simulink model "single_phase_converter_i_pr_closeloop"  (R2022b)
settings: Solver=VariableStepAuto  StartTime=0.0  StopTime=0.1  FixedStep=1e-6  MaxStep=1e-8  RelTol=1e-7
model workspace (MAT data in the model file):
  Kp = 0.2
  Kr = 10
  Ts = 2.5e-05
  wc = 6.28318530718
  wr = 314.159265359
libraries: spsMosfetLib x4, spsSeriesRLCBranchLib x4, spsCurrentMeasurementLib x1, spsDCVoltageSourceLib x1, spsIdealSwitchLib x1, simulink x1, dspsigops x1, sps_lib x1
settings Model: Creator=SSC  LastModifiedBy=SSC

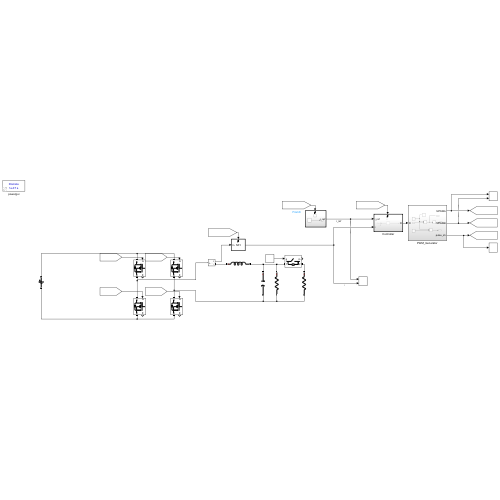
[thumbnail: Simulink's stored preview of the top-level diagram]
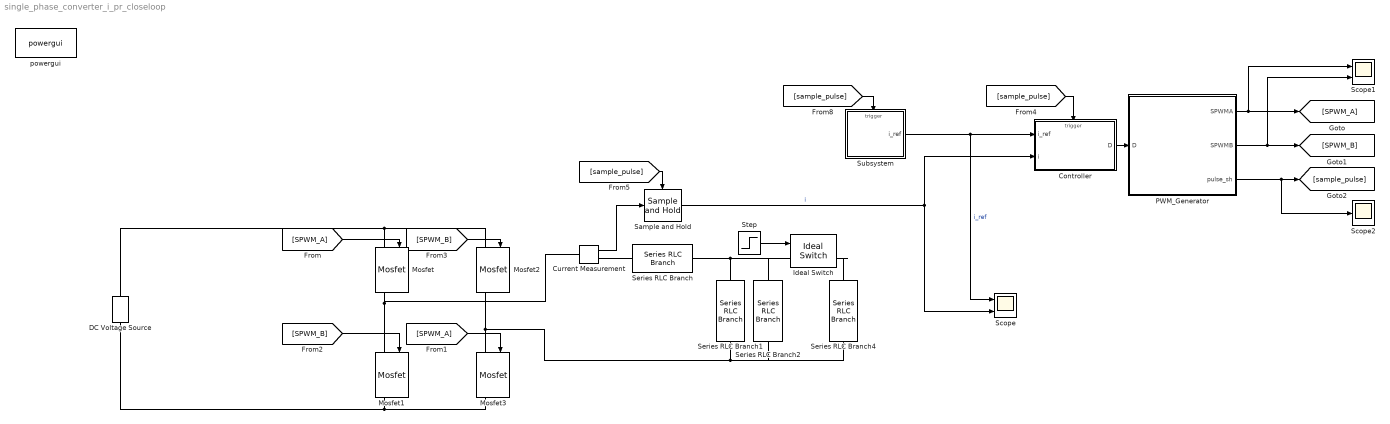
== system single_phase_converter_i_pr_closeloop ==
  Controller : Subsystem
  Current Measurement : spsCurrentMeasurementLib/Current Measurement  PhasorSimulation=off  OutputType=Complex  PSBequivalent=0
  DC Voltage Source : spsDCVoltageSourceLib/DC Voltage Source  Amplitude=48  Measurements=None
  Ideal Switch : spsIdealSwitchLib/Ideal Switch  Ron=1e-5  Lon=0  IC=0  Rs=1e5  Cs=inf  Measurements=on
  Mosfet{,1..3} (4 alike) : spsMosfetLib/Mosfet  Ron=0.1  Lon=0  Rd=0.01  Vfd=0  IC=0  Rs=1e5  Cs=inf  Measurements=on
  PWM_Generator : Subsystem
  Sample and Hold : dspsigops/Sample and Hold  trig=Rising edge  initCond=0  latchinput=off
  Scope : Scope  NumInputPorts=2
  Scope1 : Scope  NumInputPorts=2
  Scope2 : Scope
  Series RLC Branch : spsSeriesRLCBranchLib/Series RLC Branch  LConnTagsString=__new0  RConnTagsString=__new0  BranchType=L  Resistance=1  Inductance=2e-3  SetiL0=off  InitialCurrent=0  Capacitance=1e-6  Setx0=off  InitialVoltage=0  Measurements=None
  Series RLC Branch1 : spsSeriesRLCBranchLib/Series RLC Branch  LConnTagsString=__new0  RConnTagsString=__new0  BranchType=C  Resistance=1  Inductance=1e-3  SetiL0=off  InitialCurrent=0  Capacitance=25e-6  Setx0=off  InitialVoltage=0  Measurements=None
  Series RLC Branch2 : spsSeriesRLCBranchLib/Series RLC Branch  LConnTagsString=__new0  RConnTagsString=__new0  BranchType=R  Resistance=12  Inductance=1e-3  SetiL0=off  InitialCurrent=0  Capacitance=1e-6  Setx0=off  InitialVoltage=0  Measurements=None
  Series RLC Branch4 : spsSeriesRLCBranchLib/Series RLC Branch  LConnTagsString=__new0  RConnTagsString=__new0  BranchType=R  Resistance=12  Inductance=1e-3  SetiL0=off  InitialCurrent=0  Capacitance=1e-6  Setx0=off  InitialVoltage=0  Measurements=None
  Step : Step  Time=0.05  SampleTime=0
  Subsystem : Subsystem
  powergui : sps_lib/powergui  Priority=1  SimulationMode=Discrete  SampleTime=1e-7  frequency=60  Iterations=50  frequencyindice=0  Pbase=100e6  ErrMax=1e-4  UnitsV=kV  UnitsW=MW  buscounter=0  FunctionMessages=off  echomessages=off  EnableUseOfTLC=off  CurrentSourceSwitches=off  DisableSnubberDevices=off  DisableRonSwitches=off  DisableVfSwitches=off  DisplayEquations=off  AutomaticDiscreteSolvers=off  SolverType=Tustin/Backward Euler (TBE)  Interpol=off  ExternalGateDelay=off  methode=off  Ts=100  x0status=blocks  SPID=on  SwTol=0  HookPort=off  NonlinearTolerance=1e-4  nMaxIteration=100  ContinueOnMaxIteration=off  RestoreLinks=warning  ResistiveCurrentMeasurement=off  Frange=[0:2:500]  Ylog=off  Xlog=on  ShowGrid=off  save=off  variable=ZData  structure=0  ZoomFFT=off  StartTime=0.0  cycles=1  DisplayStyle=1  fundamental=60  FreqAxis=off  MaxFrequency=1000  frequencyindicesteady=1  RmsSteady=1  display=off
  wires:
  Sample and Hold/1 -> Scope/2, Controller/2(i)  "i"
  [SPWM_A] -> Mosfet/1
  [SPWM_A] -> Mosfet3/1
  [SPWM_B] -> Mosfet1/1
  [SPWM_B] -> Mosfet2/1
  PWM_Generator/1(SPWMA) -> [SPWM_A], Scope1/1
  PWM_Generator/2(SPWMB) -> [SPWM_B], Scope1/2
  Controller/1(D) -> PWM_Generator/1(D)
  PWM_Generator/3(pulse_sh) -> Scope2/1, [sample_pulse]
  Subsystem/1(i_ref) -> Scope/1, Controller/1(i_ref)  "i_ref"
  [sample_pulse] -> Controller/Trigger
  [sample_pulse] -> Subsystem/Trigger
  Step/1 -> Ideal Switch/1
  Current Measurement/1 -> Sample and Hold/1
  [sample_pulse] -> Sample and Hold/Trigger
  connections:
  Series RLC Branch/RConn1 -- Series RLC Branch2/LConn1 -- Ideal Switch/LConn1 -- Series RLC Branch1/LConn1
  Mosfet1/LConn1 -- Current Measurement/LConn1 -- Mosfet/RConn1
  Mosfet/LConn1 -- Mosfet2/LConn1 -- DC Voltage Source/RConn1
  DC Voltage Source/LConn1 -- Mosfet3/RConn1 -- Mosfet1/RConn1
  Mosfet3/LConn1 -- Mosfet2/RConn1 -- Series RLC Branch2/RConn1 -- Series RLC Branch4/RConn1 -- Series RLC Branch1/RConn1
  Ideal Switch/RConn1 -- Series RLC Branch4/LConn1
  Current Measurement/RConn1 -- Series RLC Branch/LConn1

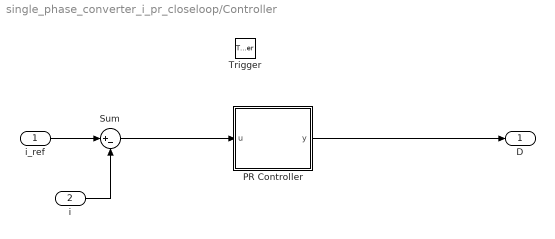
== system single_phase_converter_i_pr_closeloop/Controller ==
  i_ref : Inport
  i : Inport  Port=2
  Trigger : TriggerPort  VariantControl=(inherit)
  PR Controller : Subsystem
  Sum : Sum  Inputs=|+-
  D : Outport
  wires:
  i/1 -> Sum/2
  Sum/1 -> PR Controller/1(u)
  i_ref/1 -> Sum/1
  PR Controller/1(y) -> D/1

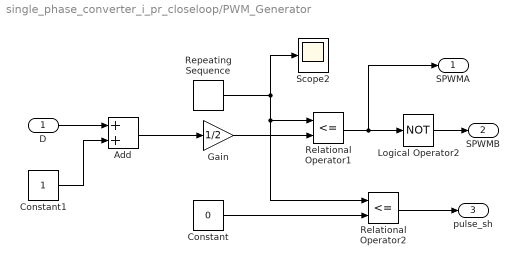
== system single_phase_converter_i_pr_closeloop/PWM_Generator ==
  D : Inport
  Add : Sum
  Constant : Constant  Value=0
  Constant1 : Constant
  Gain : Gain  Gain=1/2
  Logical Operator2 : Logic  Operator=NOT  AllPortsSameDT=off  OutDataTypeStr=boolean
  Relational Operator1 : RelationalOperator  Operator=<=  OutDataTypeStr=boolean  RndMeth=Simplest  InputSameDT=off
  Relational Operator2 : RelationalOperator  Operator=<=  OutDataTypeStr=boolean  RndMeth=Simplest  InputSameDT=off
  Repeating Sequence : simulink/Sources/Repeating Sequence  rep_seq_t=[0 0.125e-4 0.25e-4]  rep_seq_y=[0 1 0]
  Scope2 : Scope
  SPWMA : Outport
  SPWMB : Outport  Port=2
  pulse_sh : Outport  Port=3
  wires:
  Relational Operator1/1 -> SPWMA/1, Logical Operator2/1
  Logical Operator2/1 -> SPWMB/1
  Repeating Sequence/1 -> Relational Operator2/1, Relational Operator1/1, Scope2/1
  Relational Operator2/1 -> pulse_sh/1
  Constant/1 -> Relational Operator2/2
  Add/1 -> Gain/1
  D/1 -> Add/1
  Gain/1 -> Relational Operator1/2
  Constant1/1 -> Add/2

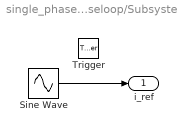
== system single_phase_converter_i_pr_closeloop/Subsystem ==
  Trigger : TriggerPort  VariantControl=(inherit)
  Sine Wave : Sin  Amplitude=2*sqrt(2)  Frequency=50*2*pi
  i_ref : Outport
  wires:
  Sine Wave/1 -> i_ref/1

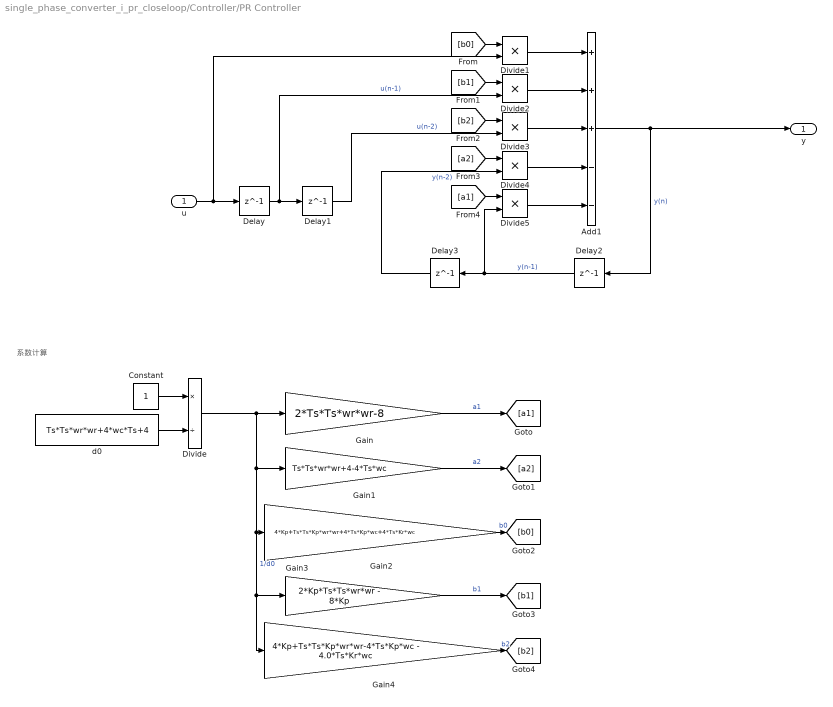
== system single_phase_converter_i_pr_closeloop/Controller/PR Controller ==
  note: 系数计算
  u : Inport
  Add1 : Sum  Inputs=+++--
  Constant : Constant
  Delay{,1..3} (4 alike) : Delay  DelayLength=1  InitialCondition=0
  Divide : Product  Inputs=*/
  Divide{1..5} (5 alike) : Product  Inputs=**
  Gain : Gain  Gain=2*Ts*Ts*wr*wr-8
  Gain1 : Gain  Gain=Ts*Ts*wr*wr+4-4*Ts*wc
  Gain2 : Gain  Gain=4*Kp+Ts*Ts*Kp*wr*wr+4*Ts*Kp*wc+4*Ts*Kr*wc
  Gain3 : Gain  Gain=2*Kp*Ts*Ts*wr*wr - 8*Kp
  Gain4 : Gain  Gain=4*Kp+Ts*Ts*Kp*wr*wr-4*Ts*Kp*wc - 4.0*Ts*Kr*wc
  d0 : Constant  Value=Ts*Ts*wr*wr+4*wc*Ts+4
  y : Outport
  wires:
  u/1 -> Delay/1, Divide1/2
  Constant/1 -> Divide/1
  d0/1 -> Divide/2
  Divide/1 -> Gain4/1, Gain3/1, Gain2/1, Gain1/1, Gain/1  "1/d0"
  Gain/1 -> [a1]  "a1"
  Gain1/1 -> [a2]  "a2"
  Gain2/1 -> [b0]  "b0"
  Gain3/1 -> [b1]  "b1"
  Gain4/1 -> [b2]  "b2"
  Divide1/1 -> Add1/1
  [b0] -> Divide1/1
  Delay/1 -> Delay1/1, Divide2/2  "u(n-1)"
  Delay1/1 -> Divide3/2  "u(n-2)"
  [b1] -> Divide2/1
  [b2] -> Divide3/1
  Divide2/1 -> Add1/2
  Divide3/1 -> Add1/3
  Add1/1 -> y/1, Delay2/1  "y(n)"
  Delay2/1 -> Delay3/1, Divide5/2  "y(n-1)"
  Delay3/1 -> Divide4/2  "y(n-2)"
  Divide4/1 -> Add1/4
  Divide5/1 -> Add1/5
  [a2] -> Divide4/1
  [a1] -> Divide5/1
